simulink library "teste_lib"  (R2013a)
settings: Solver=ode45  StartTime=0.0  StopTime=10.0  RelTol=1e-3
settings Model: Creator=michelr  LastModifiedBy=michelr

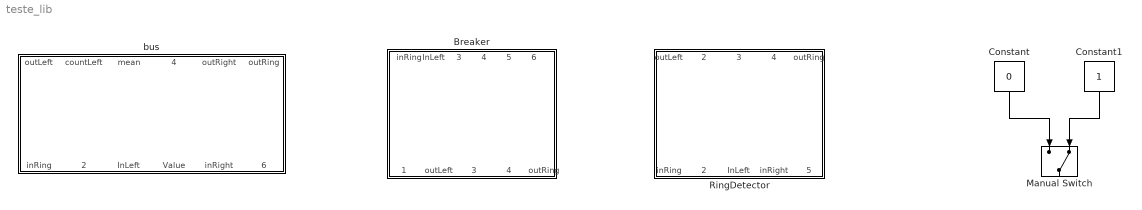
== system teste_lib ==
  Breaker : Subsystem
      settings: MinAlgLoopOccurrences=on
  Constant : Constant  RequirementInfo="{}  %GIDa_98905a27_8150_4fae_af13_32d4d819a670"  Value=0
  Constant1 : Constant
  Manual Switch : ManualSwitch  RequirementInfo="{}  %GIDa_17466918_1005_4f06_b4c1_b3de017b21cf"  CurrentSetting=0
  RingDetector : Subsystem  TreatAsAtomicUnit=on
      settings: MinAlgLoopOccurrences=on
  bus : Subsystem
      settings: MinAlgLoopOccurrences=on
  wires:
  Constant/1 -> Manual Switch/1
  Constant1/1 -> Manual Switch/2

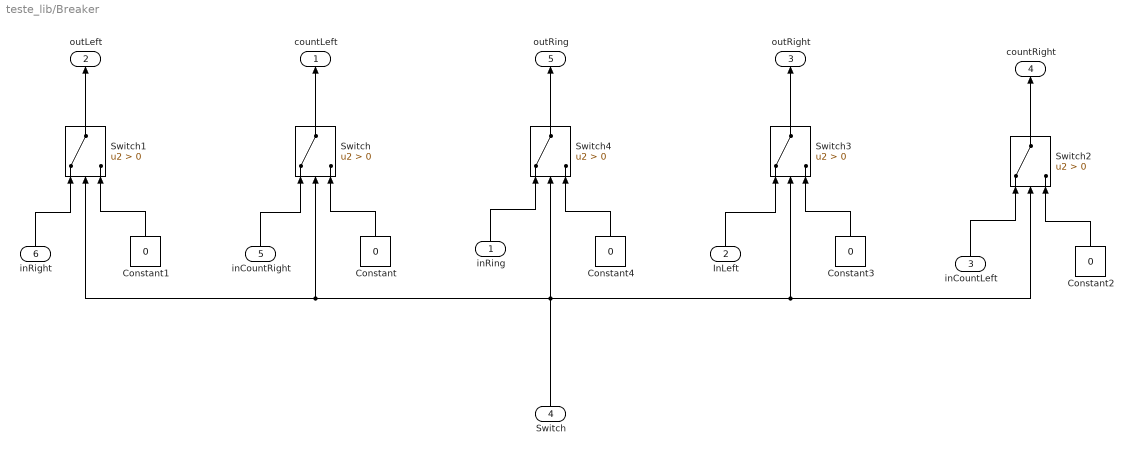
== system teste_lib/Breaker ==
  inRing : Inport
  InLeft : Inport  Port=2
  "inCountLeft " : Inport  Port=3
  "Switch " : Inport  Port=4
  inCountRight : Inport  Port=5
  inRight : Inport  Port=6
  Constant{,1..4} (5 alike) : Constant  Value=0
  Switch{,1..4} (5 alike) : Switch  Criteria=u2 > Threshold
  countLeft : Outport
  outLeft : Outport  Port=2
  outRight : Outport  Port=3
  countRight : Outport  Port=4
  outRing : Outport  Port=5
  wires:
  "inCountLeft "/1 -> Switch2/1
  Switch2/1 -> countRight/1
  Switch3/1 -> outRight/1
  InLeft/1 -> Switch3/1
  Constant3/1 -> Switch3/3
  Constant2/1 -> Switch2/3
  Switch1/1 -> outLeft/1
  inRight/1 -> Switch1/1
  Constant1/1 -> Switch1/3
  Constant/1 -> Switch/3
  Switch/1 -> countLeft/1
  inCountRight/1 -> Switch/1
  "Switch "/1 -> Switch4/2, Switch1/2, Switch/2, Switch3/2, Switch2/2
  inRing/1 -> Switch4/1
  Constant4/1 -> Switch4/3
  Switch4/1 -> outRing/1

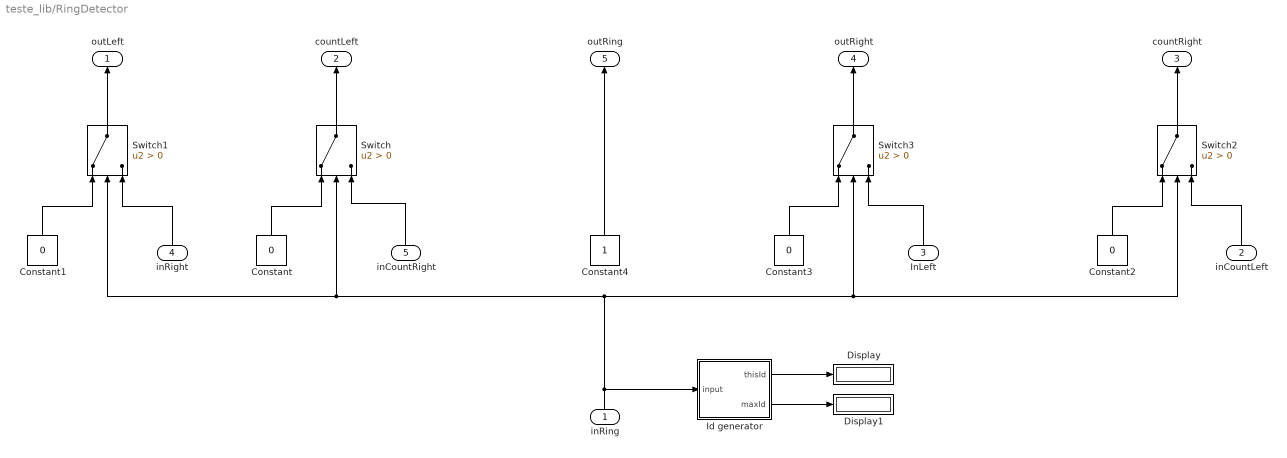
== system teste_lib/RingDetector ==
  inRing : Inport
  "inCountLeft " : Inport  Port=2
  InLeft : Inport  Port=3
  inRight : Inport  Port=4
  inCountRight : Inport  Port=5
  Constant{,1..3} (4 alike) : Constant  Value=0
  Constant4 : Constant
  Display : Display
  Display1 : Display
  Id generator : MATLAB Function  TreatAsAtomicUnit=on
  Switch{,1..3} (4 alike) : Switch  Criteria=u2 > Threshold
  outLeft : Outport
  countLeft : Outport  Port=2
  countRight : Outport  Port=3
  outRight : Outport  Port=4
  outRing : Outport  Port=5
  wires:
  "inCountLeft "/1 -> Switch2/3
  Constant2/1 -> Switch2/1
  InLeft/1 -> Switch3/3
  Constant3/1 -> Switch3/1
  inCountRight/1 -> Switch/3
  Constant/1 -> Switch/1
  Constant1/1 -> Switch1/1
  inRight/1 -> Switch1/3
  inRing/1 -> Id generator/1(input), Switch/2, Switch1/2, Switch3/2, Switch2/2
  Switch2/1 -> countRight/1
  Switch3/1 -> outRight/1
  Switch1/1 -> outLeft/1
  Switch/1 -> countLeft/1
  Id generator/2(maxId) -> Display1/1
  Id generator/1(thisId) -> Display/1
  Constant4/1 -> outRing/1

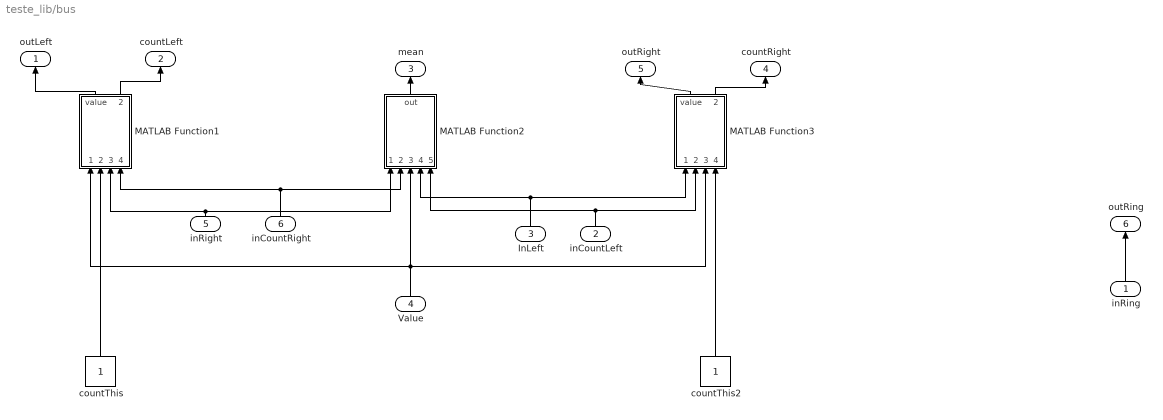
== system teste_lib/bus ==
  inRing : Inport
  "inCountLeft " : Inport  Port=2
  InLeft : Inport  Port=3
  Value : Inport  Port=4
  inRight : Inport  Port=5
  inCountRight : Inport  Port=6
  MATLAB Function1 : MATLAB Function  TreatAsAtomicUnit=on
  MATLAB Function2 : MATLAB Function  TreatAsAtomicUnit=on
  MATLAB Function3 : MATLAB Function  TreatAsAtomicUnit=on
  countThis : Constant
  countThis2 : Constant
  outLeft : Outport
  countLeft : Outport  Port=2
  mean : Outport  Port=3
  countRight : Outport  Port=4
  outRight : Outport  Port=5
  outRing : Outport  Port=6
  wires:
  countThis/1 -> MATLAB Function1/2(count1)
  countThis2/1 -> MATLAB Function3/4(count2)
  Value/1 -> MATLAB Function2/3(in2), MATLAB Function1/1(in1), MATLAB Function3/3(in2)
  inCountRight/1 -> MATLAB Function2/2(number1), MATLAB Function1/4(count2)
  inRight/1 -> MATLAB Function1/3(in2), MATLAB Function2/1(in1)
  "inCountLeft "/1 -> MATLAB Function3/2(count1), MATLAB Function2/5(number3)
  InLeft/1 -> MATLAB Function2/4(in3), MATLAB Function3/1(in1)
  MATLAB Function3/2(count) -> countRight/1
  MATLAB Function1/1(value) -> outLeft/1
  MATLAB Function1/2(count) -> countLeft/1
  MATLAB Function2/1(out) -> mean/1
  MATLAB Function3/1(value) -> outRight/1
  inRing/1 -> outRing/1

== matlab function teste_lib/RingDetector/Id generator ==
  data: thisId output; input input; maxId output
function [thisId,maxId] = fcn(input)
coder.extrinsic('gcs')
coder.extrinsic('get_param')
thisId = 0;
maxId = 0;
disp(gcs)

thisId = get_param(gcs,'Handle');
maxId = max(thisId,input);
end

== matlab function teste_lib/bus/MATLAB Function1 ==
  data: in1 input; count1 input; value output; in2 input; count2 input; count output
function [value,count] = fcn(in1,count1,in2,count2)
count = 0;
value = 0;
if count1 > 0
    count = count + count1;
    value = value + in1;
end
    
if count2 > 0
    count = count + count2;
    value = value + in2;
end

end

== matlab function teste_lib/bus/MATLAB Function2 ==
  data: in1 input; number1 input; out output; in2 input; in3 input; number3 input
function out  = fcn(in1,number1,in2,in3,number3)
count = 1;
out = in2;

if number1 > 0
    out = out + in1;
    count = count + number1;
end
if number3 > 0
    out = out + in3;
    count = count + number3;
end

out = out / count;
end

== matlab function teste_lib/bus/MATLAB Function3 ==
  data: in1 input; count1 input; value output; in2 input; count2 input; count output
function [value,count] = fcn(in1,count1,in2,count2)
count = 0;
value = 0;
if count1 > 0
    count = count + count1;
    value = value + in1;
end
    
if count2 > 0
    count = count + count2;
    value = value + in2;
end

end
